simulink model "Helikopter_new_LQI"  (R2015a)
settings: Solver=ode5  SolverMode=SingleTasking  StartTime=0.0  StopTime=Inf  FixedStep=0.001  RelTol=1e-3  AbsTol=1e-6
values from neighbouring files (symbols this model uses):
  K_lqi = lqi(lin_sys, Q, R, N)    [Helicopter_main_test.m]
  L = place(lin_A.', lin_C.', lambda).'    [Helicopter_main.m]    (also in Helicopter_main_test.m)
  lin_A = [0 1 0;     a/J_v*cos(lin_alpha_v-alpha_0) -f_v/J_v polyval(lin_M_V_diff, lin_w_v)/J_v;     0 0 -polyval(lin_U_V_diff, lin_w_v)/I_v]    [Helicopter_main.m]    (also in Helicopter_main_test.m)
  lin_alpha_v = 0    [Helicopter_main.m]    (also in Helicopter_main_test.m)
  lin_B = [0; 0; 1/I_v]    [Helicopter_main.m]    (also in Helicopter_main_test.m)
  lin_C = [1 0 0]    [Helicopter_main.m]    (also in Helicopter_main_test.m)
  lin_u_v = polyval(wsp_U_V, lin_w_v)    [Helicopter_main.m]    (also in Helicopter_main_test.m)
  lin_w_v = real(lin_w_v(lin_w_v>-50 & lin_w_v<50 & imag(lin_w_v)==0))    [Helicopter_main.m]    (also in Helicopter_main_test.m = real(lin_w_v(lin_w_v>-350 & lin_w_v<350 & imag(lin_w_v)==0)))
  wsp_V = polyfit(vp, napiecie, 1)    [Helicopter_main.m]    (also in Helicopter_main_test.m)
undefined symbols (not defined in the file): RTDAC4PCIBaseAddress
libraries: simulink x3
settings Model: SimulationMode=external  ExtModeTrigDuration=120000  ExtModeTrigLevel=0.400000  Creator=jims  LastModifiedBy=Student
settings DataIOCC: ExternalInput=[]  InitialState=[]  LimitDataPoints=off  MaxDataPoints=5000  SignalLoggingSaveFormat=ModelDataLogs  SaveOutput=off  SaveTime=off  SignalLoggingName=sigsOut
settings OptimizationCC: BooleanDataType=off  ExpressionDepthLimit=2147483647  InitFltsAndDblsToZero=on
settings DebuggingCC: SaveWithParameterizedLinksMsg=none  UnderspecifiedInitializationDetection=Classic  MergeDetectMultiDrivingBlocksExec=none  SignalResolutionControl=TryResolveAllWithWarning  MultiTaskDSMMsg=warning  MultiTaskCondExecSysMsg=none  IntegerOverflowMsg=none  FcnCallInpInsideContextMsg=UseLocalSettings  StateNameClashWarn=warning  IntegerSaturationMsg=none
settings HardwareCC: ProdBitPerLong=64  ProdBitPerPointer=64  ProdIntDivRoundTo=Zero  ProdEndianess=LittleEndian  ProdWordSize=64  ProdHWDeviceType=Intel->x86-64  TargetBitPerLong=64  TargetBitPerPointer=64  TargetIntDivRoundTo=Zero  TargetEndianess=LittleEndian  TargetWordSize=64  TargetHWDeviceType=Intel->x86-64
settings RTWCC: SystemTargetFile=rtwin.tlc  TemplateMakefile=RTDAC_win.tmf  Description=Real-Time Windows Target
settings RTWinTargetCC: TargetPreCompLibLocation=C:\Program Files\MATLAB\R2015aSP1\toolbox\sldrt\lib\win64  ModelReferenceCompliant=off  CompOptLevelCompliant=off

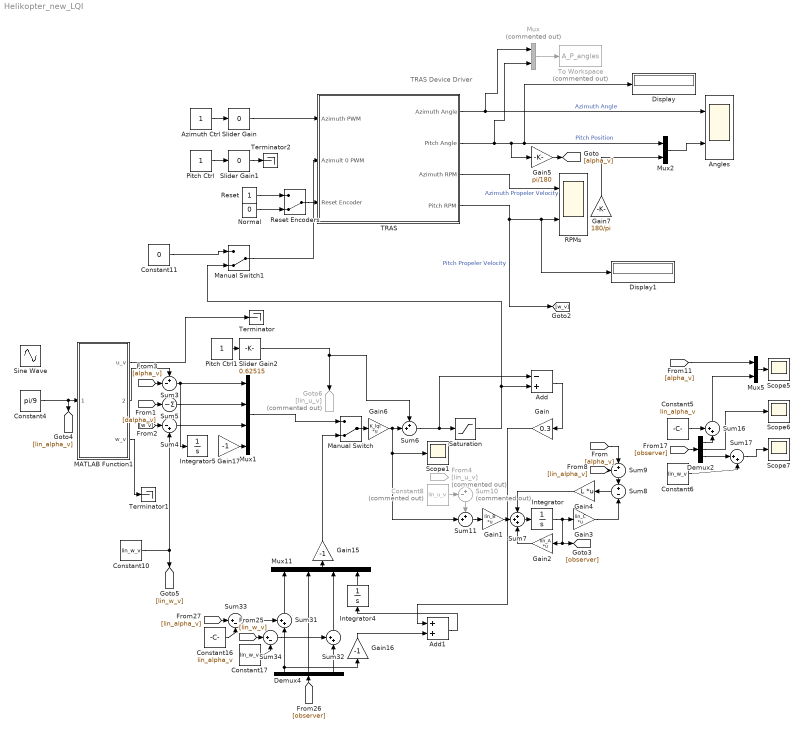
== system Helikopter_new_LQI ==
  note: TRAS Device Driver
  Add : Sum  Inputs=-+
  Add1 : Sum
  Angles : Scope  NumInputPorts=2
      settings: TimeRange=30  YMin=-6.32813~-30  YMax=-6.32812~25  SaveName=SD1  MaxDataPoints=12000
  Azimuth Ctrl : Constant  SampleTime=-1
  Constant10 : Constant  Value=lin_w_v
  Constant11 : Constant  Value=0
  Constant16 : Constant  Value=lin_alpha_v
  Constant17 : Constant  Value=lin_w_v
  Constant4 : Constant  Value=pi/9
  Constant5 : Constant  Value=lin_alpha_v
  Constant6 : Constant  Value=lin_w_v
  Constant8 : Constant  Commented=on  Value=lin_u_v
  Demux2 : Demux  Outputs=3
  Demux4 : Demux  Outputs=3
  Display : Display
  Display1 : Display
  From4 : From  Commented=on  GotoTag=lin_u_v
  Gain : Gain  Gain=0.3
  Gain1 : Gain  Gain=lin_B  Multiplication=Matrix(K*u)
  Gain15 : Gain  Gain=-1
  Gain16 : Gain  Gain=-1
  Gain17 : Gain  Gain=-1
  Gain2 : Gain  Gain=lin_A  Multiplication=Matrix(K*u)
  Gain3 : Gain  Gain=lin_C  Multiplication=Matrix(K*u)
  Gain4 : Gain  Gain=L  Multiplication=Matrix(K*u)
  Gain5 : Gain  Gain=pi/180
  Gain6 : Gain  Gain=K_lqi  Multiplication=Matrix(K*u)
  Gain7 : Gain  Gain=180/pi
  Goto6 : Goto  Commented=on  GotoTag=lin_u_v
  Integrator : Integrator  InitialCondition=[0;0;0]
  Integrator4 : Integrator
  Integrator5 : Integrator
  MATLAB Function1 : MATLAB Function  TreatAsAtomicUnit=on
  Manual Switch : ManualSwitch  CurrentSetting=0
  Manual Switch1 : ManualSwitch  CurrentSetting=0
  Mux : Mux  Commented=on  Inputs=2
  Mux1 : Mux
  Mux11 : Mux
  Mux2 : Mux  Inputs=2
  Mux5 : Mux  Inputs=2
  Normal : Constant  Value=0
  Pitch Ctrl : Constant  SampleTime=-1
  Pitch Ctrl1 : Constant  SampleTime=-1
  RPMs : Scope  NumInputPorts=2
      settings: TimeRange=30  YMin=-0.005~-0.7  YMax=0.005~0  SaveName=SD  MaxDataPoints=12000
  Reset : Constant
  Reset Encoders : ManualSwitch  CurrentSetting=0
  Saturation : Saturate  UpperLimit=1  LowerLimit=-1
  Scope{1,5..7} (4 alike) : Scope
      Scope1 settings: YMin=-0.02014  YMax=0.06521
      Scope5 settings: YMin=-0.05  YMax=0.6  SaveName=kat
      Scope6 settings: YMin=-0.18  YMax=0  SaveName=pred
      Scope7 settings: YMin=-25  YMax=250  SaveName=v_motor
  Sine Wave : Sin  Amplitude=pi/18  Frequency=0.1*pi  SampleTime=0
  Slider Gain : simulink/Math Operations/Slider Gain  low=-1  gain=0  high=1
  Slider Gain1 : simulink/Math Operations/Slider Gain  low=-1  gain=0  high=1
  Slider Gain2 : simulink/Math Operations/Slider Gain  low=-1  gain=0.62515  high=1
  Sum10 : Sum  Commented=on  Inputs=-+|
  Sum{6,11,16,31..32} (5 alike) : Sum  Inputs=++|
  Sum17 : Sum  Inputs=|++
  Sum3 : Sum  Inputs=+-|
  Sum33 : Sum  Inputs=|+-
  Sum34 : Sum  Inputs=|+-
  Sum4 : Sum  Inputs=|-+
  Sum5 : Sum  Inputs=|-|
  Sum7 : Sum  Inputs=+++
  Sum8 : Sum  Inputs=+|-
  Sum9 : Sum  Inputs=-+|
  TRAS : Subsystem  mask{BaseAddress=RTDAC4PCIBaseAddress, T0=0.001}
      mask prompts: BaseAddress "Base Address:"; T0 "Sampling Period:"
      mask Display: image(imread('TRAS.JPG'))
  Terminator : Terminator
  Terminator1 : Terminator
  Terminator2 : Terminator
  To Workspace : ToWorkspace  Commented=on  VariableName=A_P_angles  SampleTime=-1
  wires:
  TRAS/1(Azimuth Angle) -> Mux/1, Angles/1  "Azimuth Angle"
  TRAS/2(Pitch Angle) -> Mux/2, Gain5/1, Display/1, Mux2/1  "Pitch Position"
  Azimuth Ctrl/1 -> Slider Gain/1
  TRAS/3(Azimuth RPM) -> RPMs/1  "Azimuth Propeler Velocity"
  TRAS/4(Pitch RPM) -> [w_v], Display1/1, RPMs/2  "Pitch Propeler Velocity"
  Normal/1 -> Reset Encoders/2
  Reset/1 -> Reset Encoders/1
  Reset Encoders/1 -> TRAS/3(Reset Encoder)
  Pitch Ctrl/1 -> Slider Gain1/1
  Slider Gain/1 -> TRAS/1(Azimuth PWM)
  Mux/1 -> To Workspace/1
  Sum6/1 -> Add/1, Saturation/1
  Gain1/1 -> Sum7/2
  Sum7/1 -> Integrator/1
  Gain2/1 -> Sum7/3
  Integrator/1 -> Gain3/1, [observer], Gain2/1
  Gain3/1 -> Sum8/2
  Sum8/1 -> Gain4/1
  Gain4/1 -> Sum7/1
  Gain6/1 -> Sum11/2, Scope1/1, Sum6/2
  Sum9/1 -> Sum8/1
  [lin_alpha_v] -> Sum9/1
  Manual Switch/1 -> Gain6/1
  Gain15/1 -> Manual Switch/2
  Sum16/1 -> Mux5/2
  Sum17/1 -> Scope7/1
  Demux2/3 -> Sum17/1
  Mux5/1 -> Scope5/1
  Demux2/1 -> Sum16/2
  [observer] -> Demux2/1
  Constant6/1 -> Sum17/2
  Demux2/2 -> Scope6/1
  Constant5/1 -> Sum16/1
  [alpha_v] -> Mux5/1
  Sum11/1 -> Gain1/1
  Sum10/1 -> Sum11/1
  Constant8/1 -> Sum10/1
  Slider Gain2/1 -> Goto6/1, Sum6/1
  Constant10/1 -> [lin_w_v], Sum4/2
  Slider Gain1/1 -> Terminator2/1
  Constant11/1 -> Manual Switch1/1
  Manual Switch1/1 -> TRAS/2(Azimult 0 PWM)
  Saturation/1 -> Add/2, Manual Switch1/2
  [alpha_v] -> Sum9/2
  Gain5/1 -> [alpha_v]
  Pitch Ctrl1/1 -> Slider Gain2/1
  Demux4/3 -> Sum32/2
  Demux4/2 -> Mux11/2
  Demux4/1 -> Gain16/1, Sum31/2
  Integrator4/1 -> Mux11/4
  [observer] -> Demux4/1
  Mux11/1 -> Gain15/1
  Sum31/1 -> Mux11/1
  Sum32/1 -> Mux11/3
  [lin_alpha_v] -> Sum33/1
  Sum33/1 -> Sum31/1
  Constant16/1 -> Sum33/2
  Sum34/1 -> Sum32/1
  [lin_w_v] -> Sum34/1
  Constant17/1 -> Sum34/2
  [alpha_v] -> Sum3/2
  Sum3/1 -> Mux1/1, Integrator5/1
  MATLAB Function1/2(alpha_v) -> Sum3/1
  Sum4/1 -> Mux1/3
  [w_v] -> Sum4/1
  [dalpha_v] -> Sum5/1
  Sum5/1 -> Mux1/2
  MATLAB Function1/1(u_v) -> Terminator/1
  Mux1/1 -> Manual Switch/1
  MATLAB Function1/3(w_v) -> Terminator1/1
  Gain17/1 -> Mux1/4
  Add/1 -> Gain/1
  Gain16/1 -> Add1/2
  Gain/1 -> Add1/1
  Add1/1 -> Integrator4/1
  Mux2/1 -> Angles/2
  Gain7/1 -> Mux2/2
  Constant4/1 -> [lin_alpha_v], MATLAB Function1/1(alpha_vin)

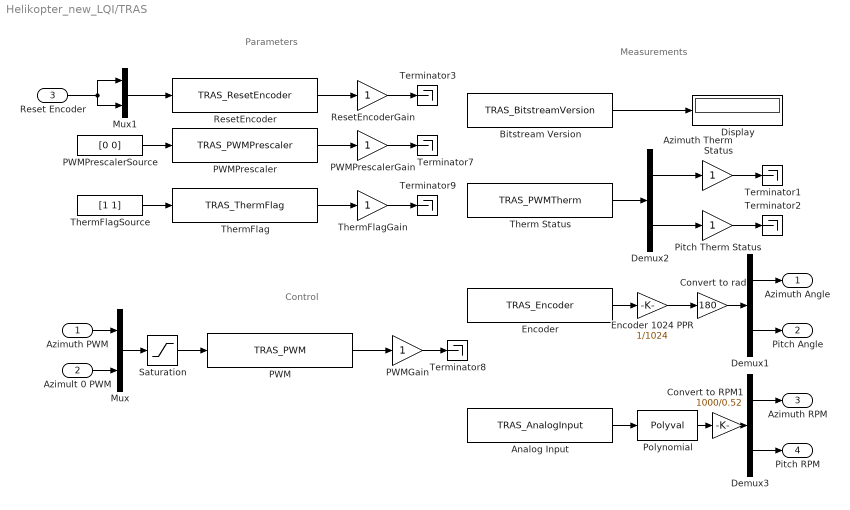
== system Helikopter_new_LQI/TRAS ==
  note: Parameters
  note: Control
  note: Measurements
  Azimuth PWM : Inport
  Azimult 0 PWM : Inport  Port=2
  Reset Encoder : Inport  Port=3
  Analog Input : S-Function  FunctionName=TRAS_AnalogInput  Parameters=BaseAddress, [1 0], [1 1], T0
  Azimuth Therm Status : Gain  SaturateOnIntegerOverflow=on  OutDataTypeStr=Inherit: Same as input  ParamDataTypeStr=Inherit: Same as input
  Bitstream Version : S-Function  FunctionName=TRAS_BitstreamVersion  Parameters=BaseAddress, T0
  Convert to RPM1 : Gain  Gain=1000/0.52  SaturateOnIntegerOverflow=on  OutDataTypeStr=Inherit: Same as input  ParamDataTypeStr=Inherit: Same as input
  Convert to rad : Gain  Gain=180  SaturateOnIntegerOverflow=on  OutDataTypeStr=Inherit: Same as input  ParamDataTypeStr=Inherit: Same as input
  Demux1 : Demux  Outputs=2
  Demux2 : Demux  Outputs=2
  Demux3 : Demux  Outputs=2
  Display : Display
  Encoder : S-Function  FunctionName=TRAS_Encoder  Parameters=BaseAddress, T0
  Encoder 1024 PPR : Gain  Gain=1/1024  SaturateOnIntegerOverflow=on  OutDataTypeStr=Inherit: Same as input  ParamDataTypeStr=Inherit: Same as input
  Mux : Mux  Inputs=2
  Mux1 : Mux  Inputs=2
  PWM : S-Function  FunctionName=TRAS_PWM  Parameters=BaseAddress, T0
  PWMGain : Gain  SaturateOnIntegerOverflow=on  OutDataTypeStr=Inherit: Same as input  ParamDataTypeStr=Inherit: Same as input
  PWMPrescaler : S-Function  FunctionName=TRAS_PWMPrescaler  Parameters=BaseAddress, T0
  PWMPrescalerGain : Gain  SaturateOnIntegerOverflow=on  OutDataTypeStr=Inherit: Same as input  ParamDataTypeStr=Inherit: Same as input
  PWMPrescalerSource : Constant  Value=[0 0]
  Pitch Therm Status : Gain  SaturateOnIntegerOverflow=on  OutDataTypeStr=Inherit: Same as input  ParamDataTypeStr=Inherit: Same as input
  Polynomial : Polyval  Coefs=wsp_V
  ResetEncoder : S-Function  FunctionName=TRAS_ResetEncoder  Parameters=BaseAddress, T0
  ResetEncoderGain : Gain  SaturateOnIntegerOverflow=on  OutDataTypeStr=Inherit: Same as input  ParamDataTypeStr=Inherit: Same as input
  Saturation : Saturate  UpperLimit=1  LowerLimit=-1
  Terminator{1..3,7..9} (6 alike) : Terminator
  Therm Status : S-Function  FunctionName=TRAS_PWMTherm  Parameters=BaseAddress, T0
  "ThermFlag " : S-Function  FunctionName=TRAS_ThermFlag  Parameters=BaseAddress, T0
  ThermFlagGain : Gain  SaturateOnIntegerOverflow=on  OutDataTypeStr=Inherit: Same as input  ParamDataTypeStr=Inherit: Same as input
  ThermFlagSource : Constant  Value=[1 1]
  Azimuth Angle : Outport  InitialOutput=0
  Pitch Angle : Outport  Port=2  InitialOutput=0
  Azimuth RPM : Outport  Port=3  InitialOutput=0
  Pitch RPM : Outport  Port=4  InitialOutput=0
  wires:
  Encoder 1024 PPR/1 -> Convert to rad/1
  Encoder/1 -> Encoder 1024 PPR/1
  Saturation/1 -> PWM/1
  Mux/1 -> Saturation/1
  PWM/1 -> PWMGain/1
  PWMGain/1 -> Terminator8/1
  ResetEncoder/1 -> ResetEncoderGain/1
  PWMPrescaler/1 -> PWMPrescalerGain/1
  Mux1/1 -> ResetEncoder/1
  PWMPrescalerSource/1 -> PWMPrescaler/1
  ResetEncoderGain/1 -> Terminator3/1
  PWMPrescalerGain/1 -> Terminator7/1
  Azimult 0 PWM/1 -> Mux/2
  Azimuth PWM/1 -> Mux/1
  Demux1/2 -> Pitch Angle/1
  Convert to rad/1 -> Demux1/1
  Demux1/1 -> Azimuth Angle/1
  Therm Status/1 -> Demux2/1
  Demux2/2 -> Pitch Therm Status/1
  Demux2/1 -> Azimuth Therm Status/1
  Azimuth Therm Status/1 -> Terminator1/1
  Pitch Therm Status/1 -> Terminator2/1
  Bitstream Version/1 -> Display/1
  Demux3/2 -> Pitch RPM/1
  Demux3/1 -> Azimuth RPM/1
  Reset Encoder/1 -> Mux1/1, Mux1/2
  Convert to RPM1/1 -> Demux3/1
  "ThermFlag "/1 -> ThermFlagGain/1
  ThermFlagSource/1 -> "ThermFlag "/1
  ThermFlagGain/1 -> Terminator9/1
  Polynomial/1 -> Convert to RPM1/1
  Analog Input/1 -> Polynomial/1

== matlab function Helikopter_new_LQI/MATLAB Function1 ==
  data: u_v output double size=1 [0..1]; alpha_v output; w_v output double size=1; alpha_vin input
function [u_v, alpha_v, w_v] = Lin(alpha_vin)

% const = load('Lin_simulink_test.mat');

a =-0.3068;
alpha_0 =-0.5223;
wsp_M_V = [-2.51456949125462e-14 2.95925329869355e-12 8.13117134030781e-09 5.04070403383922e-07 0.000115101236471819 0.000278330284083194];
wsp_U_V = [-7.44181518744928e-14 1.36310866400028e-11 2.62321306545200e-08 -6.60540818890857e-07 0.00136720921128478 0.00715086768057620];   

w_v = roots(wsp_M_V+[zeros(1,length(wsp_M_V)-1) a*sin(alpha_vin-alpha_0)]);
w_v = real(w_v(w_v>-350 & w_v<350 & imag(w_v)==0));
w_v = w_v(1);
u_v = polyval(wsp_U_V, w_v);
u_v = u_v(1);
alpha_v = alpha_vin;
